simulink model "MJAUV_Maneuverability_model_V2"  (R2022b)
settings: Solver=ode4  StartTime=0.0  StopTime=50  FixedStep=0.0001  RelTol=1e-3  EnableMultiTasking=on
libraries: sharedutil x64, matrix_library x35
(part 3 of 5)

== system MJAUV_Maneuverability_model_V2/MJ-AUV Model & PropulsionSystem/Dynamics and Kinematics/Subsystem8/Damping forces1 ==
  nu_F : Inport
  Abs : Abs
  Create Diagonal Matrix : matrix_library/Create Diagonal Matrix
  Gain : Gain  Gain=-1
  Linear Damping Matrix : Constant  Value=DL
  Matrix Multiply : Product  Multiplication=Matrix(*)
  Product : Product  SaturateOnIntegerOverflow=on  OutDataTypeStr=Inherit: Same as first input
  Quadratic Damping Vector : Constant  Value=dQ_F
  Reshape1 : Reshape  OutputDimensionality=Column vector (2-D)
  Reshape2 : Reshape  OutputDimensionality=Column vector (2-D)  OutputDimensions=[6,6]
  Sum1 : Sum  Inputs=|++  SaturateOnIntegerOverflow=on
  D * nu_F : Outport  VectorParamsAs1DForOutWhenUnconnected=off
  wires:
  Reshape2/1 -> Product/1
  Reshape1/1 -> Matrix Multiply/2, Abs/1
  nu_F/1 -> Reshape1/1
  Linear Damping Matrix/1 -> Sum1/1
  Create Diagonal Matrix/1 -> Sum1/2
  Product/1 -> Create Diagonal Matrix/1
  Abs/1 -> Product/2  "abs(nu_F)"
  Quadratic Damping Vector/1 -> Reshape2/1  "dQ"
  Matrix Multiply/1 -> D * nu_F/1
  Sum1/1 -> Gain/1  "D"
  Gain/1 -> Matrix Multiply/1

== system MJAUV_Maneuverability_model_V2/MJ-AUV Model & PropulsionSystem/Dynamics and Kinematics/Subsystem8/Restoring forces1 ==
  eta_E : Inport
  3x3 Cross Product : sharedutil/3x3 Cross Product  aMode=aMode
  3x3 Cross Product1 : sharedutil/3x3 Cross Product  aMode=aMode
  E1(e) : Subsystem
  Gain : Gain  Gain=-1  SaturateOnIntegerOverflow=on  OutDataTypeStr=Inherit: Same as input  ParamDataTypeStr=Inherit: Same as input
  Matrix Multiply : Product  Multiplication=Matrix(*)
  Matrix Multiply1 : Product  Multiplication=Matrix(*)
  Mux : Mux  Inputs=2
  Selector : Selector  InputPortWidth=7  IndexOptions=Index vector (dialog)  Indices=[4 5 6 7]  OutputSizes=1
  Sum1 : Sum  Inputs=|++  SaturateOnIntegerOverflow=on
  Sum2 : Sum  Inputs=|++  SaturateOnIntegerOverflow=on
  Transpose : Math  Operator=transpose  SignedPower=on
  fBF_E : Constant  Value=[0;0;-B_F]
  fGF_E : Constant  Value=[0;0;W_F]
  rB_F : Constant  Value=rB_F
  rG_F : Constant  Value=rG_F
  g(eta_E)_T : Outport  VectorParamsAs1DForOutWhenUnconnected=off
  wires:
  E1(e)/1(E1) -> Transpose/1  "E1(e)"
  Transpose/1 -> Matrix Multiply/1, Matrix Multiply1/1  "E1(e)^T"
  fGF_E/1 -> Matrix Multiply/2
  fBF_E/1 -> Matrix Multiply1/2
  Matrix Multiply/1 -> Sum1/1, 3x3 Cross Product/2  "fG_F"
  Matrix Multiply1/1 -> Sum1/2, 3x3 Cross Product1/2  "fB_F"
  rG_F/1 -> 3x3 Cross Product/1
  Sum1/1 -> Mux/1  "fG_F + fB_F"
  3x3 Cross Product/1 -> Sum2/1  "rG_F x fG_F"
  3x3 Cross Product1/1 -> Sum2/2  "rB_F x fG_F"
  rB_F/1 -> 3x3 Cross Product1/1
  Sum2/1 -> Mux/2
  Mux/1 -> Gain/1
  Gain/1 -> g(eta_E)_T/1
  Selector/1 -> E1(e)/1(e)  "e"
  eta_E/1 -> Selector/1  "E1(e)"

== system MJAUV_Maneuverability_model_V2/MJ-AUV Model & PropulsionSystem/Dynamics and Kinematics/Subsystem8/Rigid-body Coriolis and centripetal matrix1 ==
  nu_F : Inport
  Gain : Gain  Gain=mF  SaturateOnIntegerOverflow=on  OutDataTypeStr=Inherit: Same as input  ParamDataTypeStr=Inherit: Same as input
  Gain1 : Gain  Gain=-mF  SaturateOnIntegerOverflow=on  OutDataTypeStr=Inherit: Same as input  ParamDataTypeStr=Inherit: Same as input
  Gain2 : Gain  Gain=-1  SaturateOnIntegerOverflow=on  OutDataTypeStr=Inherit: Same as input  ParamDataTypeStr=Inherit: Same as input
  Ib_F : Subsystem
  Matrix Concatenation : Concatenate  Mode=Multidimensional array
  Matrix Concatenation1 : Concatenate  Mode=Multidimensional array
  Matrix Concatenation2 : Concatenate  Mode=Multidimensional array  ConcatenateDimension=2
  Matrix Multiply : Product  Multiplication=Matrix(*)
  Matrix Multiply1 : Product  Multiplication=Matrix(*)
  Matrix Multiply2 : Product  Multiplication=Matrix(*)
  Selector : Selector  InputPortWidth=6  IndexOptions=Index vector (dialog)  Indices=[4 5 6]  OutputSizes=1
  Selector1 : Selector  InputPortWidth=6  IndexOptions=Index vector (dialog)  Indices=[1 2 3]  OutputSizes=1
  "Skew Symmetrical Operator " : Subsystem
  Skew Symmetrical Operator : Subsystem
  "Skew Symmetrical Operator " : Subsystem
  "Skew Symmetrical Operator  " : Subsystem
  Sum1 : Sum  Inputs=|++  SaturateOnIntegerOverflow=on
  Sum2 : Sum  Inputs=|-+  SaturateOnIntegerOverflow=on
  Zero matrix (3 x 3) : Constant  Value=zeros(3,3)
  rG_F : Constant  Value=rG_F
  CRB_F : Outport  VectorParamsAs1DForOutWhenUnconnected=off
  wires:
  Gain2/1 -> Matrix Concatenation1/2  "CRB(2,2)"
  Gain/1 -> Matrix Concatenation/2  "CRB(2,1)"
  rG_F/1 -> Ib_F/1(rG_F), "Skew Symmetrical Operator  "/1(v)  "rG_F"
  "Skew Symmetrical Operator "/1(S(V)) -> Gain2/1  "S(IO * nu_F2)"
  Selector1/1 -> Skew Symmetrical Operator/1(v)  "nu_F1"
  nu_F/1 -> Selector/1, Selector1/1
  Matrix Concatenation2/1 -> CRB_F/1
  Skew Symmetrical Operator/1(S(V)) -> Sum2/1, Sum1/1  "S(nu_F1)"
  Gain1/1 -> Matrix Concatenation1/1  "CRB(1,2)"
  Zero matrix (3 x 3)/1 -> Matrix Concatenation/1  "CRB(1,1)"
  Matrix Multiply2/1 -> "Skew Symmetrical Operator "/1(v)  "IO * nu_F2"
  Sum2/1 -> Gain/1
  Matrix Concatenation1/1 -> Matrix Concatenation2/2
  Selector/1 -> "Skew Symmetrical Operator "/1(v), Matrix Multiply2/2  "nu_F2"
  Matrix Multiply/1 -> Sum2/2  "S(rG_F) * S(nu_F2)"
  Ib_F/1(Ib_F) -> Matrix Multiply2/1
  Matrix Concatenation/1 -> Matrix Concatenation2/1
  "Skew Symmetrical Operator "/1(S(V)) -> Matrix Multiply/2, Matrix Multiply1/1  "S(nu_F2)"
  Sum1/1 -> Gain1/1
  Matrix Multiply1/1 -> Sum1/2  "S(nu_F2) * S(rG_F)"
  "Skew Symmetrical Operator  "/1(S(V)) -> Matrix Multiply/1, Matrix Multiply1/2  "S(rG_F)"

== system MJAUV_Maneuverability_model_V2/MJ-AUV Model & PropulsionSystem/Dynamics and Kinematics/Subsystem8/Subsystem1 ==
  eta_E_B : Inport
  Theta : Inport  Port=2
  Demux : Demux  Outputs=3
  Mux : Mux  Inputs=3
  Mux1 : Mux  Inputs=2
  Quaternion normalisation : Subsystem
  Quaternions to Euler Angles : Subsystem
  Selector : Selector  InputPortWidth=7  IndexOptions=Index vector (dialog)  Indices=[4 5 6 7]  OutputSizes=1
  Selector1 : Selector  InputPortWidth=3  IndexOptions=Index vector (dialog)  Indices=[1]  OutputSizes=1
  Selector2 : Selector  InputPortWidth=7  IndexOptions=Index vector (dialog)  Indices=[1 2 3]  OutputSizes=1
  Selector3 : Selector  InputPortWidth=3  IndexOptions=Index vector (dialog)  Indices=[2]  OutputSizes=1
  Selector4 : Selector  InputPortWidth=3  IndexOptions=Index vector (dialog)  Indices=[3]  OutputSizes=1
  Subsystem : Subsystem
  Subsystem1 : Subsystem
  Sum : Sum  Inputs=|||++++
  eta_E_T : Outport
  wires:
  eta_E_B/1 -> Selector2/1, Selector/1
  Selector/1 -> Quaternions to Euler Angles/1(Quaternions)  "e"
  Demux/2 -> Mux/2
  Demux/3 -> Sum/1
  Quaternions to Euler Angles/1(Euler Angles) -> Demux/1
  Subsystem/1(Quaternions) -> Mux1/2
  Selector1/1 -> Sum/2  "Theta1"
  Selector2/1 -> Mux1/1  "e"
  Mux/1 -> Subsystem/1("Euler Angles ")
  Demux/1 -> Mux/1
  Mux1/1 -> Quaternion normalisation/1(eta_E)
  Sum/1 -> Subsystem1/1(In2)
  Quaternion normalisation/1(eta_E (norm)) -> eta_E_T/1
  Theta/1 -> Selector4/1, Selector3/1, Selector1/1
  Selector3/1 -> Sum/3  "Theta2"
  Selector4/1 -> Sum/4  "Theta3"
  Subsystem1/1(Out1) -> Mux/3

== system MJAUV_Maneuverability_model_V2/MJ-AUV Model & PropulsionSystem/Dynamics and Kinematics/Subsystem9/M_B ==
  Add : Sum
  Constant1 : Constant  Value=rG_B
  Subsystem : Subsystem
  Subsystem1 : Subsystem
  M_B : Outport  VectorParamsAs1DForOutWhenUnconnected=off
  wires:
  Constant1/1 -> Subsystem1/1(rG_B)
  Subsystem1/1(MRB_B) -> Add/1
  Subsystem/1(MA_B) -> Add/2
  Add/1 -> M_B/1  "M_B"

== system MJAUV_Maneuverability_model_V2/MJ-AUV Model & PropulsionSystem/Dynamics and Kinematics/Subsystem9/M_F ==
  Add : Sum
  Constant1 : Constant  Value=rG_F
  Subsystem : Subsystem
  Subsystem1 : Subsystem
  M_F : Outport  VectorParamsAs1DForOutWhenUnconnected=off
  wires:
  Constant1/1 -> Subsystem1/1(rG_F)
  Subsystem1/1(MRB_F) -> Add/1
  Subsystem/1(MA_F) -> Add/2
  Add/1 -> M_F/1  "M_F"

== system MJAUV_Maneuverability_model_V2/MJ-AUV Model & PropulsionSystem/Dynamics and Kinematics/Subsystem9/M_S ==
  rG_S : Inport
  Add : Sum
  Subsystem : Subsystem
  Subsystem1 : Subsystem
  M_S : Outport  VectorParamsAs1DForOutWhenUnconnected=off
  wires:
  Add/1 -> M_S/1  "M_S"
  Subsystem/1(MA_S) -> Add/2
  Subsystem1/1(MRB_S) -> Add/1
  rG_S/1 -> Subsystem1/1(rG_S)

== system MJAUV_Maneuverability_model_V2/MJ-AUV Model & PropulsionSystem/Dynamics and Kinematics/Subsystem9/M_T ==
  Add : Sum
  Constant1 : Constant  Value=rG_T
  Subsystem : Subsystem
  Subsystem1 : Subsystem
  M_T : Outport  VectorParamsAs1DForOutWhenUnconnected=off
  wires:
  Add/1 -> M_T/1  "M_T"
  Subsystem/1(MA_T) -> Add/2
  Subsystem1/1(MRB_T) -> Add/1
  Constant1/1 -> Subsystem1/1(rG_T)

== system MJAUV_Maneuverability_model_V2/MJ-AUV Model & PropulsionSystem/Dynamics and Kinematics/Subsystem9/Subsystem5 ==
  Theta : Inport
  K : Subsystem
  K_B : Subsystem
  K_T : Subsystem
  Selector2 : Selector  InputPortWidth=3  IndexOptions=Index vector (dialog)  Indices=[1]  OutputSizes=1
  Selector3 : Selector  InputPortWidth=3  IndexOptions=Index vector (dialog)  Indices=[2]  OutputSizes=1
  Selector6 : Selector  InputPortWidth=3  IndexOptions=Index vector (dialog)  Indices=[3]  OutputSizes=1
  Transpose1 : matrix_library/Transpose
  Transpose2 : matrix_library/Transpose
  Transpose3 : matrix_library/Transpose
  "{B}->{S} Transformation" : Subsystem
  "{S}->{T} Transformation" : Subsystem
  "{T}->{F} Transformation" : Subsystem
  K_FT : Outport
  K_TS : Outport  Port=2
  K_SB : Outport  Port=3
  wires:
  Theta/1 -> Selector2/1, Selector3/1, Selector6/1
  K/1(K_FT) -> K_FT/1
  "{B}->{S} Transformation"/1(R(v)) -> Transpose3/1  "R_BS"
  Selector6/1 -> "{T}->{F} Transformation"/1(v)
  "{T}->{F} Transformation"/1(R(v)) -> Transpose1/1  "R_TF"
  Transpose3/1 -> K_B/1(R_SB)
  "{S}->{T} Transformation"/1(R(v)) -> Transpose2/1  "R_ST"
  Transpose2/1 -> K_T/1(R_TS)
  Selector2/1 -> "{B}->{S} Transformation"/1(v)
  Transpose1/1 -> K/1(R_FT)
  Selector3/1 -> "{S}->{T} Transformation"/1(v)
  K_B/1(K_SB) -> K_SB/1
  K_T/1(K_TS) -> K_TS/1

== system MJAUV_Maneuverability_model_V2/MJ-AUV Model & PropulsionSystem/Dynamics and Kinematics/6 DOF transformation/E1(e)/Skew Symmetrical Operator ==
  v : Inport
  Constant : Constant  Value=0
  Create 3x3 Matrix : sharedutil/Create 3x3 Matrix  aMode=aMode
  Demux : Demux  Outputs=3
      settings: DisplayOption=none
  Gain : Gain  Gain=-1  SaturateOnIntegerOverflow=on  OutDataTypeStr=Inherit: Same as input  ParamDataTypeStr=Inherit: Same as input
  Gain1 : Gain  Gain=-1  SaturateOnIntegerOverflow=on  OutDataTypeStr=Inherit: Same as input  ParamDataTypeStr=Inherit: Same as input
  Gain2 : Gain  Gain=-1  SaturateOnIntegerOverflow=on  OutDataTypeStr=Inherit: Same as input  ParamDataTypeStr=Inherit: Same as input
  S(V) : Outport  VectorParamsAs1DForOutWhenUnconnected=off
  wires:
  v/1 -> Demux/1
  Create 3x3 Matrix/1 -> S(V)/1
  Gain2/1 -> Create 3x3 Matrix/2  "-v(3)"
  Gain1/1 -> Create 3x3 Matrix/7  "-v(2)"
  Gain/1 -> Create 3x3 Matrix/6  "-v(1)"
  Demux/3 -> Create 3x3 Matrix/4, Gain2/1  "v(3)"
  Demux/2 -> Create 3x3 Matrix/3, Gain1/1  "v(2)"
  Demux/1 -> Create 3x3 Matrix/8, Gain/1  "v(1)"
  Constant/1 -> Create 3x3 Matrix/5, Create 3x3 Matrix/9, Create 3x3 Matrix/1

== system MJAUV_Maneuverability_model_V2/MJ-AUV Model & PropulsionSystem/Dynamics and Kinematics/6 DOF transformation/E2(e)/Skew Symmetrical Operator ==
  v : Inport
  Constant : Constant  Value=0
  Create 3x3 Matrix : sharedutil/Create 3x3 Matrix  aMode=aMode
  Demux : Demux  Outputs=3
      settings: DisplayOption=none
  Gain : Gain  Gain=-1  SaturateOnIntegerOverflow=on  OutDataTypeStr=Inherit: Same as input  ParamDataTypeStr=Inherit: Same as input
  Gain1 : Gain  Gain=-1  SaturateOnIntegerOverflow=on  OutDataTypeStr=Inherit: Same as input  ParamDataTypeStr=Inherit: Same as input
  Gain2 : Gain  Gain=-1  SaturateOnIntegerOverflow=on  OutDataTypeStr=Inherit: Same as input  ParamDataTypeStr=Inherit: Same as input
  S(V) : Outport  VectorParamsAs1DForOutWhenUnconnected=off
  wires:
  Constant/1 -> Create 3x3 Matrix/1, Create 3x3 Matrix/9, Create 3x3 Matrix/5
  Demux/1 -> Gain/1, Create 3x3 Matrix/8  "v(1)"
  Demux/2 -> Gain1/1, Create 3x3 Matrix/3  "v(2)"
  Demux/3 -> Gain2/1, Create 3x3 Matrix/4  "v(3)"
  Gain/1 -> Create 3x3 Matrix/6  "-v(1)"
  Gain1/1 -> Create 3x3 Matrix/7  "-v(2)"
  Gain2/1 -> Create 3x3 Matrix/2  "-v(3)"
  Create 3x3 Matrix/1 -> S(V)/1
  v/1 -> Demux/1

== system MJAUV_Maneuverability_model_V2/MJ-AUV Model & PropulsionSystem/Dynamics and Kinematics/Subsystem1/H_BS/Skew Symmetrical Operator  ==
  v : Inport
  Constant : Constant  Value=0
  Create 3x3 Matrix : sharedutil/Create 3x3 Matrix  aMode=aMode
  Demux : Demux  Outputs=3
      settings: DisplayOption=none
  Gain : Gain  Gain=-1  SaturateOnIntegerOverflow=on  OutDataTypeStr=Inherit: Same as input  ParamDataTypeStr=Inherit: Same as input
  Gain1 : Gain  Gain=-1  SaturateOnIntegerOverflow=on  OutDataTypeStr=Inherit: Same as input  ParamDataTypeStr=Inherit: Same as input
  Gain2 : Gain  Gain=-1  SaturateOnIntegerOverflow=on  OutDataTypeStr=Inherit: Same as input  ParamDataTypeStr=Inherit: Same as input
  S(V) : Outport  VectorParamsAs1DForOutWhenUnconnected=off
  wires:
  v/1 -> Demux/1
  Create 3x3 Matrix/1 -> S(V)/1
  Gain2/1 -> Create 3x3 Matrix/2  "-v(3)"
  Gain1/1 -> Create 3x3 Matrix/7  "-v(2)"
  Gain/1 -> Create 3x3 Matrix/6  "-v(1)"
  Demux/3 -> Create 3x3 Matrix/4, Gain2/1  "v(3)"
  Demux/2 -> Create 3x3 Matrix/3, Gain1/1  "v(2)"
  Demux/1 -> Create 3x3 Matrix/8, Gain/1  "v(1)"
  Constant/1 -> Create 3x3 Matrix/5, Create 3x3 Matrix/9, Create 3x3 Matrix/1

== system MJAUV_Maneuverability_model_V2/MJ-AUV Model & PropulsionSystem/Dynamics and Kinematics/Subsystem2/H_ST/Skew Symmetrical Operator  ==
  v : Inport
  Constant : Constant  Value=0
  Create 3x3 Matrix : sharedutil/Create 3x3 Matrix  aMode=aMode
  Demux : Demux  Outputs=3
      settings: DisplayOption=none
  Gain : Gain  Gain=-1  SaturateOnIntegerOverflow=on  OutDataTypeStr=Inherit: Same as input  ParamDataTypeStr=Inherit: Same as input
  Gain1 : Gain  Gain=-1  SaturateOnIntegerOverflow=on  OutDataTypeStr=Inherit: Same as input  ParamDataTypeStr=Inherit: Same as input
  Gain2 : Gain  Gain=-1  SaturateOnIntegerOverflow=on  OutDataTypeStr=Inherit: Same as input  ParamDataTypeStr=Inherit: Same as input
  S(V) : Outport  VectorParamsAs1DForOutWhenUnconnected=off
  wires:
  v/1 -> Demux/1
  Create 3x3 Matrix/1 -> S(V)/1
  Gain2/1 -> Create 3x3 Matrix/2  "-v(3)"
  Gain1/1 -> Create 3x3 Matrix/7  "-v(2)"
  Gain/1 -> Create 3x3 Matrix/6  "-v(1)"
  Demux/3 -> Create 3x3 Matrix/4, Gain2/1  "v(3)"
  Demux/2 -> Create 3x3 Matrix/3, Gain1/1  "v(2)"
  Demux/1 -> Create 3x3 Matrix/8, Gain/1  "v(1)"
  Constant/1 -> Create 3x3 Matrix/5, Create 3x3 Matrix/9, Create 3x3 Matrix/1

== system MJAUV_Maneuverability_model_V2/MJ-AUV Model & PropulsionSystem/Dynamics and Kinematics/Subsystem3/H_TF/Skew Symmetrical Operator  ==
  v : Inport
  Constant : Constant  Value=0
  Create 3x3 Matrix : sharedutil/Create 3x3 Matrix  aMode=aMode
  Demux : Demux  Outputs=3
      settings: DisplayOption=none
  Gain : Gain  Gain=-1  SaturateOnIntegerOverflow=on  OutDataTypeStr=Inherit: Same as input  ParamDataTypeStr=Inherit: Same as input
  Gain1 : Gain  Gain=-1  SaturateOnIntegerOverflow=on  OutDataTypeStr=Inherit: Same as input  ParamDataTypeStr=Inherit: Same as input
  Gain2 : Gain  Gain=-1  SaturateOnIntegerOverflow=on  OutDataTypeStr=Inherit: Same as input  ParamDataTypeStr=Inherit: Same as input
  S(V) : Outport  VectorParamsAs1DForOutWhenUnconnected=off
  wires:
  Constant/1 -> Create 3x3 Matrix/1, Create 3x3 Matrix/9, Create 3x3 Matrix/5
  Demux/1 -> Gain/1, Create 3x3 Matrix/8  "v(1)"
  Demux/2 -> Gain1/1, Create 3x3 Matrix/3  "v(2)"
  Demux/3 -> Gain2/1, Create 3x3 Matrix/4  "v(3)"
  Gain/1 -> Create 3x3 Matrix/6  "-v(1)"
  Gain1/1 -> Create 3x3 Matrix/7  "-v(2)"
  Gain2/1 -> Create 3x3 Matrix/2  "-v(3)"
  Create 3x3 Matrix/1 -> S(V)/1
  v/1 -> Demux/1

== system MJAUV_Maneuverability_model_V2/MJ-AUV Model & PropulsionSystem/Dynamics and Kinematics/Subsystem4/Added Mass Coriolis and centripetal matrix/Skew Symmetrical Operator ==
  v : Inport
  Constant : Constant  Value=0
  Create 3x3 Matrix : sharedutil/Create 3x3 Matrix  aMode=aMode
  Demux : Demux  Outputs=3
      settings: DisplayOption=none
  Gain : Gain  Gain=-1  SaturateOnIntegerOverflow=on  OutDataTypeStr=Inherit: Same as input  ParamDataTypeStr=Inherit: Same as input
  Gain1 : Gain  Gain=-1  SaturateOnIntegerOverflow=on  OutDataTypeStr=Inherit: Same as input  ParamDataTypeStr=Inherit: Same as input
  Gain2 : Gain  Gain=-1  SaturateOnIntegerOverflow=on  OutDataTypeStr=Inherit: Same as input  ParamDataTypeStr=Inherit: Same as input
  S(V) : Outport  VectorParamsAs1DForOutWhenUnconnected=off
  wires:
  Constant/1 -> Create 3x3 Matrix/1, Create 3x3 Matrix/9, Create 3x3 Matrix/5
  Demux/1 -> Gain/1, Create 3x3 Matrix/8  "v(1)"
  Demux/2 -> Gain1/1, Create 3x3 Matrix/3  "v(2)"
  Demux/3 -> Gain2/1, Create 3x3 Matrix/4  "v(3)"
  Gain/1 -> Create 3x3 Matrix/6  "-v(1)"
  Gain1/1 -> Create 3x3 Matrix/7  "-v(2)"
  Gain2/1 -> Create 3x3 Matrix/2  "-v(3)"
  Create 3x3 Matrix/1 -> S(V)/1
  v/1 -> Demux/1

== system MJAUV_Maneuverability_model_V2/MJ-AUV Model & PropulsionSystem/Dynamics and Kinematics/Subsystem4/Added Mass Coriolis and centripetal matrix/Skew Symmetrical Operator  ==
  v : Inport
  Constant : Constant  Value=0
  Create 3x3 Matrix : sharedutil/Create 3x3 Matrix  aMode=aMode
  Demux : Demux  Outputs=3
      settings: DisplayOption=none
  Gain : Gain  Gain=-1  SaturateOnIntegerOverflow=on  OutDataTypeStr=Inherit: Same as input  ParamDataTypeStr=Inherit: Same as input
  Gain1 : Gain  Gain=-1  SaturateOnIntegerOverflow=on  OutDataTypeStr=Inherit: Same as input  ParamDataTypeStr=Inherit: Same as input
  Gain2 : Gain  Gain=-1  SaturateOnIntegerOverflow=on  OutDataTypeStr=Inherit: Same as input  ParamDataTypeStr=Inherit: Same as input
  S(V) : Outport  VectorParamsAs1DForOutWhenUnconnected=off
  wires:
  v/1 -> Demux/1
  Create 3x3 Matrix/1 -> S(V)/1
  Gain2/1 -> Create 3x3 Matrix/2  "-v(3)"
  Gain1/1 -> Create 3x3 Matrix/7  "-v(2)"
  Gain/1 -> Create 3x3 Matrix/6  "-v(1)"
  Demux/3 -> Create 3x3 Matrix/4, Gain2/1  "v(3)"
  Demux/2 -> Create 3x3 Matrix/3, Gain1/1  "v(2)"
  Demux/1 -> Create 3x3 Matrix/8, Gain/1  "v(1)"
  Constant/1 -> Create 3x3 Matrix/5, Create 3x3 Matrix/9, Create 3x3 Matrix/1

== system MJAUV_Maneuverability_model_V2/MJ-AUV Model & PropulsionSystem/Dynamics and Kinematics/Subsystem4/Added Mass Coriolis and centripetal matrix/Subsystem ==
  Create Diagonal Matrix1 : matrix_library/Create Diagonal Matrix
  K_pdot_B : Constant  Value=0
  M_qdot_B : Constant  Value=(pi*rho*R^2*LB^3)/12
  Mux : Mux  Inputs=6
  N_rdot_B : Constant  Value=(pi*rho*R^2*LB^3)/12
  Reshape1 : Reshape  OutputDimensionality=Column vector (2-D)  OutputDimensions=[6,6]
  X_udot_B : Constant  Value=0.1*mB
  Y_vdot_B : Constant  Value=pi*rho*R*R*LB
  Z_wdot_B : Constant  Value=pi*rho*R^2*LB
  MA_B : Outport
  wires:
  Create Diagonal Matrix1/1 -> MA_B/1
  K_pdot_B/1 -> Mux/4
  N_rdot_B/1 -> Mux/6
  M_qdot_B/1 -> Mux/5
  X_udot_B/1 -> Mux/1
  Y_vdot_B/1 -> Mux/2
  Reshape1/1 -> Create Diagonal Matrix1/1
  Mux/1 -> Reshape1/1
  Z_wdot_B/1 -> Mux/3

== system MJAUV_Maneuverability_model_V2/MJ-AUV Model & PropulsionSystem/Dynamics and Kinematics/Subsystem4/Restoring forces/E1(e) ==
  e : Inport
  Gain : Gain  Gain=2  SaturateOnIntegerOverflow=on  OutDataTypeStr=Inherit: Same as input  ParamDataTypeStr=Inherit: Same as input
  "Gain " : Gain  Gain=2  SaturateOnIntegerOverflow=on  OutDataTypeStr=Inherit: Same as input  ParamDataTypeStr=Inherit: Same as input
  I (3x3) : Constant  Value=eye(3)
  Matrix Multiply : Product  Multiplication=Matrix(*)
  Product : Product  SaturateOnIntegerOverflow=on  OutDataTypeStr=Inherit: Same as first input
  Selector : Selector  InputPortWidth=4  IndexOptions=Index vector (dialog)  Indices=[1]  OutputSizes=1
  Selector1 : Selector  InputPortWidth=4  IndexOptions=Index vector (dialog)  Indices=[2 3 4]  OutputSizes=1
  Skew Symmetrical Operator : Subsystem
  Sum : Sum  Inputs=+++  SaturateOnIntegerOverflow=on
  E1 : Outport  VectorParamsAs1DForOutWhenUnconnected=off
  wires:
  e/1 -> Selector/1, Selector1/1
  Selector/1 -> "Gain "/1  "eta"
  Selector1/1 -> Skew Symmetrical Operator/1(v)  "eps"
  Skew Symmetrical Operator/1(S(V)) -> Matrix Multiply/1, Matrix Multiply/2, Product/2
  Matrix Multiply/1 -> Gain/1
  "Gain "/1 -> Product/1
  I (3x3)/1 -> Sum/1
  Product/1 -> Sum/2
  Gain/1 -> Sum/3
  Sum/1 -> E1/1

== system MJAUV_Maneuverability_model_V2/MJ-AUV Model & PropulsionSystem/Dynamics and Kinematics/Subsystem4/Rigid-body Coriolis and centripetal matrix/Skew Symmetrical Operator  ==
  v : Inport
  Constant : Constant  Value=0
  Create 3x3 Matrix : sharedutil/Create 3x3 Matrix  aMode=aMode
  Demux : Demux  Outputs=3
      settings: DisplayOption=none
  Gain : Gain  Gain=-1  SaturateOnIntegerOverflow=on  OutDataTypeStr=Inherit: Same as input  ParamDataTypeStr=Inherit: Same as input
  Gain1 : Gain  Gain=-1  SaturateOnIntegerOverflow=on  OutDataTypeStr=Inherit: Same as input  ParamDataTypeStr=Inherit: Same as input
  Gain2 : Gain  Gain=-1  SaturateOnIntegerOverflow=on  OutDataTypeStr=Inherit: Same as input  ParamDataTypeStr=Inherit: Same as input
  S(V) : Outport  VectorParamsAs1DForOutWhenUnconnected=off
  wires:
  v/1 -> Demux/1
  Create 3x3 Matrix/1 -> S(V)/1
  Gain2/1 -> Create 3x3 Matrix/2  "-v(3)"
  Gain1/1 -> Create 3x3 Matrix/7  "-v(2)"
  Gain/1 -> Create 3x3 Matrix/6  "-v(1)"
  Demux/3 -> Create 3x3 Matrix/4, Gain2/1  "v(3)"
  Demux/2 -> Create 3x3 Matrix/3, Gain1/1  "v(2)"
  Demux/1 -> Create 3x3 Matrix/8, Gain/1  "v(1)"
  Constant/1 -> Create 3x3 Matrix/5, Create 3x3 Matrix/9, Create 3x3 Matrix/1

== system MJAUV_Maneuverability_model_V2/MJ-AUV Model & PropulsionSystem/Dynamics and Kinematics/Subsystem4/Rigid-body Coriolis and centripetal matrix/Skew Symmetrical Operator ==
  v : Inport
  Constant : Constant  Value=0
  Create 3x3 Matrix : sharedutil/Create 3x3 Matrix  aMode=aMode
  Demux : Demux  Outputs=3
      settings: DisplayOption=none
  Gain : Gain  Gain=-1  SaturateOnIntegerOverflow=on  OutDataTypeStr=Inherit: Same as input  ParamDataTypeStr=Inherit: Same as input
  Gain1 : Gain  Gain=-1  SaturateOnIntegerOverflow=on  OutDataTypeStr=Inherit: Same as input  ParamDataTypeStr=Inherit: Same as input
  Gain2 : Gain  Gain=-1  SaturateOnIntegerOverflow=on  OutDataTypeStr=Inherit: Same as input  ParamDataTypeStr=Inherit: Same as input
  S(V) : Outport  VectorParamsAs1DForOutWhenUnconnected=off
  wires:
  v/1 -> Demux/1
  Create 3x3 Matrix/1 -> S(V)/1
  Gain2/1 -> Create 3x3 Matrix/2  "-v(3)"
  Gain1/1 -> Create 3x3 Matrix/7  "-v(2)"
  Gain/1 -> Create 3x3 Matrix/6  "-v(1)"
  Demux/3 -> Create 3x3 Matrix/4, Gain2/1  "v(3)"
  Demux/2 -> Create 3x3 Matrix/3, Gain1/1  "v(2)"
  Demux/1 -> Create 3x3 Matrix/8, Gain/1  "v(1)"
  Constant/1 -> Create 3x3 Matrix/5, Create 3x3 Matrix/9, Create 3x3 Matrix/1

== system MJAUV_Maneuverability_model_V2/MJ-AUV Model & PropulsionSystem/Dynamics and Kinematics/Subsystem4/Rigid-body Coriolis and centripetal matrix/Skew Symmetrical Operator  ==
  v : Inport
  Constant : Constant  Value=0
  Create 3x3 Matrix : sharedutil/Create 3x3 Matrix  aMode=aMode
  Demux : Demux  Outputs=3
      settings: DisplayOption=none
  Gain : Gain  Gain=-1  SaturateOnIntegerOverflow=on  OutDataTypeStr=Inherit: Same as input  ParamDataTypeStr=Inherit: Same as input
  Gain1 : Gain  Gain=-1  SaturateOnIntegerOverflow=on  OutDataTypeStr=Inherit: Same as input  ParamDataTypeStr=Inherit: Same as input
  Gain2 : Gain  Gain=-1  SaturateOnIntegerOverflow=on  OutDataTypeStr=Inherit: Same as input  ParamDataTypeStr=Inherit: Same as input
  S(V) : Outport  VectorParamsAs1DForOutWhenUnconnected=off
  wires:
  Constant/1 -> Create 3x3 Matrix/1, Create 3x3 Matrix/9, Create 3x3 Matrix/5
  Demux/1 -> Gain/1, Create 3x3 Matrix/8  "v(1)"
  Demux/2 -> Gain1/1, Create 3x3 Matrix/3  "v(2)"
  Demux/3 -> Gain2/1, Create 3x3 Matrix/4  "v(3)"
  Gain/1 -> Create 3x3 Matrix/6  "-v(1)"
  Gain1/1 -> Create 3x3 Matrix/7  "-v(2)"
  Gain2/1 -> Create 3x3 Matrix/2  "-v(3)"
  Create 3x3 Matrix/1 -> S(V)/1
  v/1 -> Demux/1

== system MJAUV_Maneuverability_model_V2/MJ-AUV Model & PropulsionSystem/Dynamics and Kinematics/Subsystem4/Rigid-body Coriolis and centripetal matrix/Skew Symmetrical Operator   ==
  v : Inport
  Constant : Constant  Value=0
  Create 3x3 Matrix : sharedutil/Create 3x3 Matrix  aMode=aMode
  Demux : Demux  Outputs=3
      settings: DisplayOption=none
  Gain : Gain  Gain=-1  SaturateOnIntegerOverflow=on  OutDataTypeStr=Inherit: Same as input  ParamDataTypeStr=Inherit: Same as input
  Gain1 : Gain  Gain=-1  SaturateOnIntegerOverflow=on  OutDataTypeStr=Inherit: Same as input  ParamDataTypeStr=Inherit: Same as input
  Gain2 : Gain  Gain=-1  SaturateOnIntegerOverflow=on  OutDataTypeStr=Inherit: Same as input  ParamDataTypeStr=Inherit: Same as input
  S(V) : Outport  VectorParamsAs1DForOutWhenUnconnected=off
  wires:
  v/1 -> Demux/1
  Create 3x3 Matrix/1 -> S(V)/1
  Gain2/1 -> Create 3x3 Matrix/2  "-v(3)"
  Gain1/1 -> Create 3x3 Matrix/7  "-v(2)"
  Gain/1 -> Create 3x3 Matrix/6  "-v(1)"
  Demux/3 -> Create 3x3 Matrix/4, Gain2/1  "v(3)"
  Demux/2 -> Create 3x3 Matrix/3, Gain1/1  "v(2)"
  Demux/1 -> Create 3x3 Matrix/8, Gain/1  "v(1)"
  Constant/1 -> Create 3x3 Matrix/5, Create 3x3 Matrix/9, Create 3x3 Matrix/1

== system MJAUV_Maneuverability_model_V2/MJ-AUV Model & PropulsionSystem/Dynamics and Kinematics/Subsystem4/Rigid-body Coriolis and centripetal matrix/Subsystem ==
  rG_B : Inport
  Add : Sum
  Constant2 : Constant  Value=IB
  Gain5 : Gain  Gain=-mB
  Matrix Multiply4 : Product  Multiplication=Matrix(*)
  Skew Symmetrical Operator1 : Subsystem
  Ib_B : Outport
  wires:
  rG_B/1 -> Skew Symmetrical Operator1/1(v)  "rG_B"
  Constant2/1 -> Add/1
  Gain5/1 -> Add/2
  Matrix Multiply4/1 -> Gain5/1
  Skew Symmetrical Operator1/1(S(V)) -> Matrix Multiply4/1, Matrix Multiply4/2  "skewsymm(rG_B)"
  Add/1 -> Ib_B/1  "Ib_B"

== system MJAUV_Maneuverability_model_V2/MJ-AUV Model & PropulsionSystem/Dynamics and Kinematics/Subsystem5/K/Skew Symmetrical Operator  ==
  v : Inport
  Constant : Constant  Value=0
  Create 3x3 Matrix : sharedutil/Create 3x3 Matrix  aMode=aMode
  Demux : Demux  Outputs=3
      settings: DisplayOption=none
  Gain : Gain  Gain=-1  SaturateOnIntegerOverflow=on  OutDataTypeStr=Inherit: Same as input  ParamDataTypeStr=Inherit: Same as input
  Gain1 : Gain  Gain=-1  SaturateOnIntegerOverflow=on  OutDataTypeStr=Inherit: Same as input  ParamDataTypeStr=Inherit: Same as input
  Gain2 : Gain  Gain=-1  SaturateOnIntegerOverflow=on  OutDataTypeStr=Inherit: Same as input  ParamDataTypeStr=Inherit: Same as input
  S(V) : Outport  VectorParamsAs1DForOutWhenUnconnected=off
  wires:
  Constant/1 -> Create 3x3 Matrix/1, Create 3x3 Matrix/9, Create 3x3 Matrix/5
  Demux/1 -> Gain/1, Create 3x3 Matrix/8  "v(1)"
  Demux/2 -> Gain1/1, Create 3x3 Matrix/3  "v(2)"
  Demux/3 -> Gain2/1, Create 3x3 Matrix/4  "v(3)"
  Gain/1 -> Create 3x3 Matrix/6  "-v(1)"
  Gain1/1 -> Create 3x3 Matrix/7  "-v(2)"
  Gain2/1 -> Create 3x3 Matrix/2  "-v(3)"
  Create 3x3 Matrix/1 -> S(V)/1
  v/1 -> Demux/1

== system MJAUV_Maneuverability_model_V2/MJ-AUV Model & PropulsionSystem/Dynamics and Kinematics/Subsystem5/K_B/Skew Symmetrical Operator  ==
  v : Inport
  Constant : Constant  Value=0
  Create 3x3 Matrix : sharedutil/Create 3x3 Matrix  aMode=aMode
  Demux : Demux  Outputs=3
      settings: DisplayOption=none
  Gain : Gain  Gain=-1  SaturateOnIntegerOverflow=on  OutDataTypeStr=Inherit: Same as input  ParamDataTypeStr=Inherit: Same as input
  Gain1 : Gain  Gain=-1  SaturateOnIntegerOverflow=on  OutDataTypeStr=Inherit: Same as input  ParamDataTypeStr=Inherit: Same as input
  Gain2 : Gain  Gain=-1  SaturateOnIntegerOverflow=on  OutDataTypeStr=Inherit: Same as input  ParamDataTypeStr=Inherit: Same as input
  S(V) : Outport  VectorParamsAs1DForOutWhenUnconnected=off
  wires:
  v/1 -> Demux/1
  Create 3x3 Matrix/1 -> S(V)/1
  Gain2/1 -> Create 3x3 Matrix/2  "-v(3)"
  Gain1/1 -> Create 3x3 Matrix/7  "-v(2)"
  Gain/1 -> Create 3x3 Matrix/6  "-v(1)"
  Demux/3 -> Create 3x3 Matrix/4, Gain2/1  "v(3)"
  Demux/2 -> Create 3x3 Matrix/3, Gain1/1  "v(2)"
  Demux/1 -> Create 3x3 Matrix/8, Gain/1  "v(1)"
  Constant/1 -> Create 3x3 Matrix/5, Create 3x3 Matrix/9, Create 3x3 Matrix/1

== system MJAUV_Maneuverability_model_V2/MJ-AUV Model & PropulsionSystem/Dynamics and Kinematics/Subsystem5/K_T/Skew Symmetrical Operator  ==
  v : Inport
  Constant : Constant  Value=0
  Create 3x3 Matrix : sharedutil/Create 3x3 Matrix  aMode=aMode
  Demux : Demux  Outputs=3
      settings: DisplayOption=none
  Gain : Gain  Gain=-1  SaturateOnIntegerOverflow=on  OutDataTypeStr=Inherit: Same as input  ParamDataTypeStr=Inherit: Same as input
  Gain1 : Gain  Gain=-1  SaturateOnIntegerOverflow=on  OutDataTypeStr=Inherit: Same as input  ParamDataTypeStr=Inherit: Same as input
  Gain2 : Gain  Gain=-1  SaturateOnIntegerOverflow=on  OutDataTypeStr=Inherit: Same as input  ParamDataTypeStr=Inherit: Same as input
  S(V) : Outport  VectorParamsAs1DForOutWhenUnconnected=off
  wires:
  v/1 -> Demux/1
  Create 3x3 Matrix/1 -> S(V)/1
  Gain2/1 -> Create 3x3 Matrix/2  "-v(3)"
  Gain1/1 -> Create 3x3 Matrix/7  "-v(2)"
  Gain/1 -> Create 3x3 Matrix/6  "-v(1)"
  Demux/3 -> Create 3x3 Matrix/4, Gain2/1  "v(3)"
  Demux/2 -> Create 3x3 Matrix/3, Gain1/1  "v(2)"
  Demux/1 -> Create 3x3 Matrix/8, Gain/1  "v(1)"
  Constant/1 -> Create 3x3 Matrix/5, Create 3x3 Matrix/9, Create 3x3 Matrix/1

== system MJAUV_Maneuverability_model_V2/MJ-AUV Model & PropulsionSystem/Dynamics and Kinematics/Subsystem6/Added Mass Coriolis and centripetal matrix1/Skew Symmetrical Operator ==
  v : Inport
  Constant : Constant  Value=0
  Create 3x3 Matrix : sharedutil/Create 3x3 Matrix  aMode=aMode
  Demux : Demux  Outputs=3
      settings: DisplayOption=none
  Gain : Gain  Gain=-1  SaturateOnIntegerOverflow=on  OutDataTypeStr=Inherit: Same as input  ParamDataTypeStr=Inherit: Same as input
  Gain1 : Gain  Gain=-1  SaturateOnIntegerOverflow=on  OutDataTypeStr=Inherit: Same as input  ParamDataTypeStr=Inherit: Same as input
  Gain2 : Gain  Gain=-1  SaturateOnIntegerOverflow=on  OutDataTypeStr=Inherit: Same as input  ParamDataTypeStr=Inherit: Same as input
  S(V) : Outport  VectorParamsAs1DForOutWhenUnconnected=off
  wires:
  v/1 -> Demux/1
  Create 3x3 Matrix/1 -> S(V)/1
  Gain2/1 -> Create 3x3 Matrix/2  "-v(3)"
  Gain1/1 -> Create 3x3 Matrix/7  "-v(2)"
  Gain/1 -> Create 3x3 Matrix/6  "-v(1)"
  Demux/3 -> Create 3x3 Matrix/4, Gain2/1  "v(3)"
  Demux/2 -> Create 3x3 Matrix/3, Gain1/1  "v(2)"
  Demux/1 -> Create 3x3 Matrix/8, Gain/1  "v(1)"
  Constant/1 -> Create 3x3 Matrix/5, Create 3x3 Matrix/9, Create 3x3 Matrix/1

== system MJAUV_Maneuverability_model_V2/MJ-AUV Model & PropulsionSystem/Dynamics and Kinematics/Subsystem6/Added Mass Coriolis and centripetal matrix1/Skew Symmetrical Operator  ==
  v : Inport
  Constant : Constant  Value=0
  Create 3x3 Matrix : sharedutil/Create 3x3 Matrix  aMode=aMode
  Demux : Demux  Outputs=3
      settings: DisplayOption=none
  Gain : Gain  Gain=-1  SaturateOnIntegerOverflow=on  OutDataTypeStr=Inherit: Same as input  ParamDataTypeStr=Inherit: Same as input
  Gain1 : Gain  Gain=-1  SaturateOnIntegerOverflow=on  OutDataTypeStr=Inherit: Same as input  ParamDataTypeStr=Inherit: Same as input
  Gain2 : Gain  Gain=-1  SaturateOnIntegerOverflow=on  OutDataTypeStr=Inherit: Same as input  ParamDataTypeStr=Inherit: Same as input
  S(V) : Outport  VectorParamsAs1DForOutWhenUnconnected=off
  wires:
  Constant/1 -> Create 3x3 Matrix/1, Create 3x3 Matrix/9, Create 3x3 Matrix/5
  Demux/1 -> Gain/1, Create 3x3 Matrix/8  "v(1)"
  Demux/2 -> Gain1/1, Create 3x3 Matrix/3  "v(2)"
  Demux/3 -> Gain2/1, Create 3x3 Matrix/4  "v(3)"
  Gain/1 -> Create 3x3 Matrix/6  "-v(1)"
  Gain1/1 -> Create 3x3 Matrix/7  "-v(2)"
  Gain2/1 -> Create 3x3 Matrix/2  "-v(3)"
  Create 3x3 Matrix/1 -> S(V)/1
  v/1 -> Demux/1

== system MJAUV_Maneuverability_model_V2/MJ-AUV Model & PropulsionSystem/Dynamics and Kinematics/Subsystem6/Added Mass Coriolis and centripetal matrix1/Subsystem ==
  Create Diagonal Matrix1 : matrix_library/Create Diagonal Matrix
  K_pdot_S : Constant  Value=0
  M_qdot_S : Constant  Value=(pi*rho*R^2*LS^3)/12
  Mux : Mux  Inputs=6
  N_rdot_S : Constant  Value=(pi*rho*R^2*LS^3)/12
  Reshape1 : Reshape  OutputDimensionality=Column vector (2-D)  OutputDimensions=[6,6]
  X_udot_S : Constant  Value=0.1*mS
  Y_vdot_S : Constant  Value=pi*rho*R*R*LS
  Z_wdot_S : Constant  Value=pi*rho*R^2*LS
  MA_S : Outport
  wires:
  Z_wdot_S/1 -> Mux/3
  Mux/1 -> Reshape1/1
  Reshape1/1 -> Create Diagonal Matrix1/1
  Y_vdot_S/1 -> Mux/2
  X_udot_S/1 -> Mux/1
  M_qdot_S/1 -> Mux/5
  N_rdot_S/1 -> Mux/6
  K_pdot_S/1 -> Mux/4
  Create Diagonal Matrix1/1 -> MA_S/1

== system MJAUV_Maneuverability_model_V2/MJ-AUV Model & PropulsionSystem/Dynamics and Kinematics/Subsystem6/Restoring forces1/E1(e) ==
  e : Inport
  Gain : Gain  Gain=2  SaturateOnIntegerOverflow=on  OutDataTypeStr=Inherit: Same as input  ParamDataTypeStr=Inherit: Same as input
  "Gain " : Gain  Gain=2  SaturateOnIntegerOverflow=on  OutDataTypeStr=Inherit: Same as input  ParamDataTypeStr=Inherit: Same as input
  I (3x3) : Constant  Value=eye(3)
  Matrix Multiply : Product  Multiplication=Matrix(*)
  Product : Product  SaturateOnIntegerOverflow=on  OutDataTypeStr=Inherit: Same as first input
  Selector : Selector  InputPortWidth=4  IndexOptions=Index vector (dialog)  Indices=[1]  OutputSizes=1
  Selector1 : Selector  InputPortWidth=4  IndexOptions=Index vector (dialog)  Indices=[2 3 4]  OutputSizes=1
  Skew Symmetrical Operator : Subsystem
  Sum : Sum  Inputs=+++  SaturateOnIntegerOverflow=on
  E1 : Outport  VectorParamsAs1DForOutWhenUnconnected=off
  wires:
  Sum/1 -> E1/1
  Gain/1 -> Sum/3
  Product/1 -> Sum/2
  I (3x3)/1 -> Sum/1
  "Gain "/1 -> Product/1
  Matrix Multiply/1 -> Gain/1
  Skew Symmetrical Operator/1(S(V)) -> Product/2, Matrix Multiply/2, Matrix Multiply/1
  Selector1/1 -> Skew Symmetrical Operator/1(v)  "eps"
  Selector/1 -> "Gain "/1  "eta"
  e/1 -> Selector1/1, Selector/1

== system MJAUV_Maneuverability_model_V2/MJ-AUV Model & PropulsionSystem/Dynamics and Kinematics/Subsystem6/Rigid-body Coriolis and centripetal matrix1/Skew Symmetrical Operator  ==
  v : Inport
  Constant : Constant  Value=0
  Create 3x3 Matrix : sharedutil/Create 3x3 Matrix  aMode=aMode
  Demux : Demux  Outputs=3
      settings: DisplayOption=none
  Gain : Gain  Gain=-1  SaturateOnIntegerOverflow=on  OutDataTypeStr=Inherit: Same as input  ParamDataTypeStr=Inherit: Same as input
  Gain1 : Gain  Gain=-1  SaturateOnIntegerOverflow=on  OutDataTypeStr=Inherit: Same as input  ParamDataTypeStr=Inherit: Same as input
  Gain2 : Gain  Gain=-1  SaturateOnIntegerOverflow=on  OutDataTypeStr=Inherit: Same as input  ParamDataTypeStr=Inherit: Same as input
  S(V) : Outport  VectorParamsAs1DForOutWhenUnconnected=off
  wires:
  Constant/1 -> Create 3x3 Matrix/1, Create 3x3 Matrix/9, Create 3x3 Matrix/5
  Demux/1 -> Gain/1, Create 3x3 Matrix/8  "v(1)"
  Demux/2 -> Gain1/1, Create 3x3 Matrix/3  "v(2)"
  Demux/3 -> Gain2/1, Create 3x3 Matrix/4  "v(3)"
  Gain/1 -> Create 3x3 Matrix/6  "-v(1)"
  Gain1/1 -> Create 3x3 Matrix/7  "-v(2)"
  Gain2/1 -> Create 3x3 Matrix/2  "-v(3)"
  Create 3x3 Matrix/1 -> S(V)/1
  v/1 -> Demux/1

== system MJAUV_Maneuverability_model_V2/MJ-AUV Model & PropulsionSystem/Dynamics and Kinematics/Subsystem6/Rigid-body Coriolis and centripetal matrix1/Skew Symmetrical Operator ==
  v : Inport
  Constant : Constant  Value=0
  Create 3x3 Matrix : sharedutil/Create 3x3 Matrix  aMode=aMode
  Demux : Demux  Outputs=3
      settings: DisplayOption=none
  Gain : Gain  Gain=-1  SaturateOnIntegerOverflow=on  OutDataTypeStr=Inherit: Same as input  ParamDataTypeStr=Inherit: Same as input
  Gain1 : Gain  Gain=-1  SaturateOnIntegerOverflow=on  OutDataTypeStr=Inherit: Same as input  ParamDataTypeStr=Inherit: Same as input
  Gain2 : Gain  Gain=-1  SaturateOnIntegerOverflow=on  OutDataTypeStr=Inherit: Same as input  ParamDataTypeStr=Inherit: Same as input
  S(V) : Outport  VectorParamsAs1DForOutWhenUnconnected=off
  wires:
  Constant/1 -> Create 3x3 Matrix/1, Create 3x3 Matrix/9, Create 3x3 Matrix/5
  Demux/1 -> Gain/1, Create 3x3 Matrix/8  "v(1)"
  Demux/2 -> Gain1/1, Create 3x3 Matrix/3  "v(2)"
  Demux/3 -> Gain2/1, Create 3x3 Matrix/4  "v(3)"
  Gain/1 -> Create 3x3 Matrix/6  "-v(1)"
  Gain1/1 -> Create 3x3 Matrix/7  "-v(2)"
  Gain2/1 -> Create 3x3 Matrix/2  "-v(3)"
  Create 3x3 Matrix/1 -> S(V)/1
  v/1 -> Demux/1

== system MJAUV_Maneuverability_model_V2/MJ-AUV Model & PropulsionSystem/Dynamics and Kinematics/Subsystem6/Rigid-body Coriolis and centripetal matrix1/Skew Symmetrical Operator  ==
  v : Inport
  Constant : Constant  Value=0
  Create 3x3 Matrix : sharedutil/Create 3x3 Matrix  aMode=aMode
  Demux : Demux  Outputs=3
      settings: DisplayOption=none
  Gain : Gain  Gain=-1  SaturateOnIntegerOverflow=on  OutDataTypeStr=Inherit: Same as input  ParamDataTypeStr=Inherit: Same as input
  Gain1 : Gain  Gain=-1  SaturateOnIntegerOverflow=on  OutDataTypeStr=Inherit: Same as input  ParamDataTypeStr=Inherit: Same as input
  Gain2 : Gain  Gain=-1  SaturateOnIntegerOverflow=on  OutDataTypeStr=Inherit: Same as input  ParamDataTypeStr=Inherit: Same as input
  S(V) : Outport  VectorParamsAs1DForOutWhenUnconnected=off
  wires:
  v/1 -> Demux/1
  Create 3x3 Matrix/1 -> S(V)/1
  Gain2/1 -> Create 3x3 Matrix/2  "-v(3)"
  Gain1/1 -> Create 3x3 Matrix/7  "-v(2)"
  Gain/1 -> Create 3x3 Matrix/6  "-v(1)"
  Demux/3 -> Create 3x3 Matrix/4, Gain2/1  "v(3)"
  Demux/2 -> Create 3x3 Matrix/3, Gain1/1  "v(2)"
  Demux/1 -> Create 3x3 Matrix/8, Gain/1  "v(1)"
  Constant/1 -> Create 3x3 Matrix/5, Create 3x3 Matrix/9, Create 3x3 Matrix/1

== system MJAUV_Maneuverability_model_V2/MJ-AUV Model & PropulsionSystem/Dynamics and Kinematics/Subsystem6/Rigid-body Coriolis and centripetal matrix1/Skew Symmetrical Operator   ==
  v : Inport
  Constant : Constant  Value=0
  Create 3x3 Matrix : sharedutil/Create 3x3 Matrix  aMode=aMode
  Demux : Demux  Outputs=3
      settings: DisplayOption=none
  Gain : Gain  Gain=-1  SaturateOnIntegerOverflow=on  OutDataTypeStr=Inherit: Same as input  ParamDataTypeStr=Inherit: Same as input
  Gain1 : Gain  Gain=-1  SaturateOnIntegerOverflow=on  OutDataTypeStr=Inherit: Same as input  ParamDataTypeStr=Inherit: Same as input
  Gain2 : Gain  Gain=-1  SaturateOnIntegerOverflow=on  OutDataTypeStr=Inherit: Same as input  ParamDataTypeStr=Inherit: Same as input
  S(V) : Outport  VectorParamsAs1DForOutWhenUnconnected=off
  wires:
  Constant/1 -> Create 3x3 Matrix/1, Create 3x3 Matrix/9, Create 3x3 Matrix/5
  Demux/1 -> Gain/1, Create 3x3 Matrix/8  "v(1)"
  Demux/2 -> Gain1/1, Create 3x3 Matrix/3  "v(2)"
  Demux/3 -> Gain2/1, Create 3x3 Matrix/4  "v(3)"
  Gain/1 -> Create 3x3 Matrix/6  "-v(1)"
  Gain1/1 -> Create 3x3 Matrix/7  "-v(2)"
  Gain2/1 -> Create 3x3 Matrix/2  "-v(3)"
  Create 3x3 Matrix/1 -> S(V)/1
  v/1 -> Demux/1

== system MJAUV_Maneuverability_model_V2/MJ-AUV Model & PropulsionSystem/Dynamics and Kinematics/Subsystem6/Rigid-body Coriolis and centripetal matrix1/Subsystem ==
  rG_S : Inport
  Add : Sum
  Constant2 : Constant  Value=IS
  Gain5 : Gain  Gain=-mS
  Matrix Multiply4 : Product  Multiplication=Matrix(*)
  Skew Symmetrical Operator1 : Subsystem
  Ib_S : Outport
  wires:
  rG_S/1 -> Skew Symmetrical Operator1/1(v)  "rG_S"
  Constant2/1 -> Add/1
  Gain5/1 -> Add/2
  Matrix Multiply4/1 -> Gain5/1
  Skew Symmetrical Operator1/1(S(V)) -> Matrix Multiply4/1, Matrix Multiply4/2  "skewsymm(rG_S)"
  Add/1 -> Ib_S/1  "Ib_S"

== system MJAUV_Maneuverability_model_V2/MJ-AUV Model & PropulsionSystem/Dynamics and Kinematics/Subsystem6/Subsystem1/Quaternion normalisation ==
  eta_E : Inport
  Mux : Mux  Inputs=2
  Product : Product  Inputs=*/  SaturateOnIntegerOverflow=on  OutDataTypeStr=Inherit: Same as first input
  Reshape : Reshape  OutputDimensionality=Column vector (2-D)
  Selector : Selector  InputPortWidth=7  IndexOptions=Index vector (dialog)  Indices=[1 2 3]  OutputSizes=1
  Selector1 : Selector  InputPortWidth=7  IndexOptions=Index vector (dialog)  Indices=[4 5 6 7]  OutputSizes=1
  norm 1x4 vector : Subsystem
  eta_E (norm) : Outport  VectorParamsAs1DForOutWhenUnconnected=off
  wires:
  norm 1x4 vector/1(norm) -> Product/2
  Reshape/1 -> eta_E (norm)/1
  Mux/1 -> Reshape/1
  Product/1 -> Mux/2
  Selector/1 -> Mux/1
  Selector1/1 -> Product/1, norm 1x4 vector/1(Inport)
  eta_E/1 -> Selector/1, Selector1/1  "eta_E"

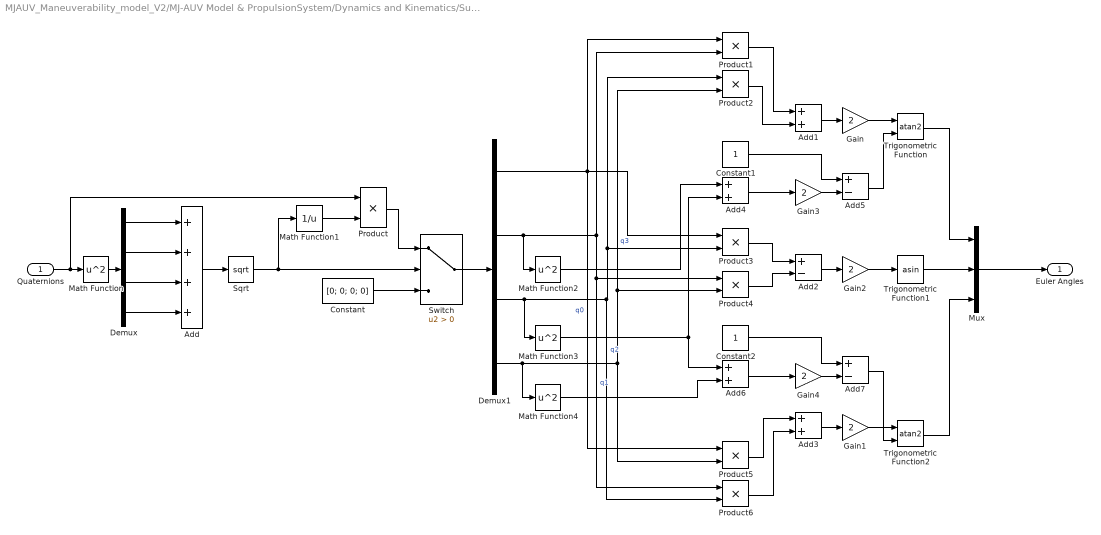
== system MJAUV_Maneuverability_model_V2/MJ-AUV Model & PropulsionSystem/Dynamics and Kinematics/Subsystem6/Subsystem1/Quaternions to Euler Angles ==
  Quaternions : Inport
  Add : Sum  Inputs=4
  Add{1,3..4,6} (4 alike) : Sum
  Add2 : Sum  Inputs=+-
  Add5 : Sum  Inputs=+-
  Add7 : Sum  Inputs=+-
  Constant : Constant  Value=[0; 0; 0; 0]
  Constant1 : Constant
  Constant2 : Constant
  Demux : Demux
  Demux1 : Demux
  Gain{,1..4} (5 alike) : Gain  Gain=2
  Math Function{,2..4} (4 alike) : Math  Operator=square  SignedPower=on
  Math Function1 : Math  Operator=reciprocal  SignedPower=on
  Mux : Mux  Inputs=3
  Product{,1..6} (7 alike) : Product
  Sqrt : Sqrt
  Switch : Switch  Criteria=u2 > Threshold  SaturateOnIntegerOverflow=off  InputSameDT=off
  Trigonometric Function : Trigonometry  Operator=atan2
  Trigonometric Function1 : Trigonometry  Operator=asin
  Trigonometric Function2 : Trigonometry  Operator=atan2
  Euler Angles : Outport  VectorParamsAs1DForOutWhenUnconnected=off
  wires:
  Quaternions/1 -> Product/1, Math Function/1
  Add/1 -> Sqrt/1
  Sqrt/1 -> Math Function1/1, Switch/2
  Constant/1 -> Switch/3
  Math Function1/1 -> Product/2
  Product/1 -> Switch/1
  Switch/1 -> Demux1/1
  Demux1/1 -> Product5/1, Product3/1, Product1/1  "q0"
  Demux1/2 -> Product6/1, Product4/1, Product1/2, Math Function2/1  "q1"
  Demux1/3 -> Product6/2, Product3/2, Product2/1, Math Function3/1  "q2"
  Demux1/4 -> Product5/2, Product4/2, Product2/2, Math Function4/1  "q3"
  Trigonometric Function1/1 -> Mux/2
  Mux/1 -> Euler Angles/1
  Trigonometric Function/1 -> Mux/1
  Trigonometric Function2/1 -> Mux/3
  Gain/1 -> Trigonometric Function/1
  Gain1/1 -> Trigonometric Function2/1
  Gain2/1 -> Trigonometric Function1/1
  Add1/1 -> Gain/1
  Add2/1 -> Gain2/1
  Add3/1 -> Gain1/1
  Product3/1 -> Add2/1
  Product4/1 -> Add2/2
  Product5/1 -> Add3/1
  Product6/1 -> Add3/2
  Product2/1 -> Add1/2
  Product1/1 -> Add1/1
  Add4/1 -> Gain3/1
  Gain3/1 -> Add5/2
  Constant1/1 -> Add5/1
  Add5/1 -> Trigonometric Function/2
  Add7/1 -> Trigonometric Function2/2
  Add6/1 -> Gain4/1
  Gain4/1 -> Add7/2
  Constant2/1 -> Add7/1
  Math Function2/1 -> Add4/1
  Math Function3/1 -> Add6/1, Add4/2
  Math Function4/1 -> Add6/2
  Demux/1 -> Add/1
  Demux/2 -> Add/2
  Demux/3 -> Add/3
  Demux/4 -> Add/4
  Math Function/1 -> Demux/1

== system MJAUV_Maneuverability_model_V2/MJ-AUV Model & PropulsionSystem/Dynamics and Kinematics/Subsystem6/Subsystem1/Subsystem ==
  "Euler Angles " : Inport
  Add : Sum
  Add1 : Sum  Inputs=-+
  Add2 : Sum
  Add3 : Sum  Inputs=+-
  Demux : Demux  Outputs=3
  Demux1 : Demux  Outputs=3
  Gain : Gain  Gain=0.5
  Mux : Mux
  Product{,1..7} (8 alike) : Product  Inputs=3
  Trigonometric Function : Trigonometry
  Trigonometric Function1 : Trigonometry  Operator=cos
  Quaternions : Outport  VectorParamsAs1DForOutWhenUnconnected=off
  wires:
  Add3/1 -> Mux/4
  Add2/1 -> Mux/3
  Add/1 -> Mux/1
  Add1/1 -> Mux/2
  Mux/1 -> Quaternions/1
  Product7/1 -> Add3/2
  Product6/1 -> Add3/1
  Product5/1 -> Add2/2
  Product4/1 -> Add2/1
  Product3/1 -> Add1/2
  Product2/1 -> Add1/1
  Product1/1 -> Add/2
  Product/1 -> Add/1
  Demux1/3 -> Product5/3, Product1/3, Product3/3, Product7/3  "cos(Y/2)"
  Demux1/1 -> Product5/1, Product2/1, Product1/1, Product6/1  "cos(R/2)"
  Demux1/2 -> Product6/2, Product1/2, Product3/2, Product4/2  "cos(P/2)"
  Trigonometric Function1/1 -> Demux1/1
  Demux/3 -> Product/3, Product2/3, Product4/3, Product6/3  "sin(Y/2)"
  Demux/2 -> Product/2, Product2/2, Product5/2, Product7/2  "sin(P/2)"
  Demux/1 -> Product/1, Product3/1, Product4/1, Product7/1  "sin(R/2)"
  Trigonometric Function/1 -> Demux/1
  Gain/1 -> Trigonometric Function/1, Trigonometric Function1/1
  "Euler Angles "/1 -> Gain/1

== system MJAUV_Maneuverability_model_V2/MJ-AUV Model & PropulsionSystem/Dynamics and Kinematics/Subsystem6/Subsystem1/Subsystem1 ==
  In2 : Inport
  Abs : Abs  SaturateOnIntegerOverflow=off
  Add : Sum  Inputs=-+
  Constant : Constant  Value=2*pi
  Switch : Switch  Criteria=u2 > Threshold  Threshold=pi  SaturateOnIntegerOverflow=off  InputSameDT=off
  Out1 : Outport
  wires:
  In2/1 -> Add/2, Switch/3, Abs/1
  Switch/1 -> Out1/1
  Add/1 -> Switch/1
  Abs/1 -> Switch/2
  Constant/1 -> Add/1

== system MJAUV_Maneuverability_model_V2/MJ-AUV Model & PropulsionSystem/Dynamics and Kinematics/Subsystem7/Added Mass Coriolis and centripetal matrix1/Skew Symmetrical Operator ==
  v : Inport
  Constant : Constant  Value=0
  Create 3x3 Matrix : sharedutil/Create 3x3 Matrix  aMode=aMode
  Demux : Demux  Outputs=3
      settings: DisplayOption=none
  Gain : Gain  Gain=-1  SaturateOnIntegerOverflow=on  OutDataTypeStr=Inherit: Same as input  ParamDataTypeStr=Inherit: Same as input
  Gain1 : Gain  Gain=-1  SaturateOnIntegerOverflow=on  OutDataTypeStr=Inherit: Same as input  ParamDataTypeStr=Inherit: Same as input
  Gain2 : Gain  Gain=-1  SaturateOnIntegerOverflow=on  OutDataTypeStr=Inherit: Same as input  ParamDataTypeStr=Inherit: Same as input
  S(V) : Outport  VectorParamsAs1DForOutWhenUnconnected=off
  wires:
  Constant/1 -> Create 3x3 Matrix/1, Create 3x3 Matrix/9, Create 3x3 Matrix/5
  Demux/1 -> Gain/1, Create 3x3 Matrix/8  "v(1)"
  Demux/2 -> Gain1/1, Create 3x3 Matrix/3  "v(2)"
  Demux/3 -> Gain2/1, Create 3x3 Matrix/4  "v(3)"
  Gain/1 -> Create 3x3 Matrix/6  "-v(1)"
  Gain1/1 -> Create 3x3 Matrix/7  "-v(2)"
  Gain2/1 -> Create 3x3 Matrix/2  "-v(3)"
  Create 3x3 Matrix/1 -> S(V)/1
  v/1 -> Demux/1

== system MJAUV_Maneuverability_model_V2/MJ-AUV Model & PropulsionSystem/Dynamics and Kinematics/Subsystem7/Added Mass Coriolis and centripetal matrix1/Skew Symmetrical Operator  ==
  v : Inport
  Constant : Constant  Value=0
  Create 3x3 Matrix : sharedutil/Create 3x3 Matrix  aMode=aMode
  Demux : Demux  Outputs=3
      settings: DisplayOption=none
  Gain : Gain  Gain=-1  SaturateOnIntegerOverflow=on  OutDataTypeStr=Inherit: Same as input  ParamDataTypeStr=Inherit: Same as input
  Gain1 : Gain  Gain=-1  SaturateOnIntegerOverflow=on  OutDataTypeStr=Inherit: Same as input  ParamDataTypeStr=Inherit: Same as input
  Gain2 : Gain  Gain=-1  SaturateOnIntegerOverflow=on  OutDataTypeStr=Inherit: Same as input  ParamDataTypeStr=Inherit: Same as input
  S(V) : Outport  VectorParamsAs1DForOutWhenUnconnected=off
  wires:
  v/1 -> Demux/1
  Create 3x3 Matrix/1 -> S(V)/1
  Gain2/1 -> Create 3x3 Matrix/2  "-v(3)"
  Gain1/1 -> Create 3x3 Matrix/7  "-v(2)"
  Gain/1 -> Create 3x3 Matrix/6  "-v(1)"
  Demux/3 -> Create 3x3 Matrix/4, Gain2/1  "v(3)"
  Demux/2 -> Create 3x3 Matrix/3, Gain1/1  "v(2)"
  Demux/1 -> Create 3x3 Matrix/8, Gain/1  "v(1)"
  Constant/1 -> Create 3x3 Matrix/5, Create 3x3 Matrix/9, Create 3x3 Matrix/1

== system MJAUV_Maneuverability_model_V2/MJ-AUV Model & PropulsionSystem/Dynamics and Kinematics/Subsystem7/Added Mass Coriolis and centripetal matrix1/Subsystem ==
  Create Diagonal Matrix1 : matrix_library/Create Diagonal Matrix
  K_pdot_T : Constant  Value=0
  M_qdot_T : Constant  Value=(pi*rho*R^2*LT^3)/12
  Mux : Mux  Inputs=6
  N_rdot_T : Constant  Value=(pi*rho*R^2*LT^3)/12
  Reshape1 : Reshape  OutputDimensionality=Column vector (2-D)  OutputDimensions=[6,6]
  X_udot_T : Constant  Value=0.1*mT
  Y_vdot_T : Constant  Value=pi*rho*R*R*LT
  Z_wdot_T : Constant  Value=pi*rho*R^2*LT
  MA_T : Outport
  wires:
  Z_wdot_T/1 -> Mux/3
  Mux/1 -> Reshape1/1
  Reshape1/1 -> Create Diagonal Matrix1/1
  Y_vdot_T/1 -> Mux/2
  X_udot_T/1 -> Mux/1
  M_qdot_T/1 -> Mux/5
  N_rdot_T/1 -> Mux/6
  K_pdot_T/1 -> Mux/4
  Create Diagonal Matrix1/1 -> MA_T/1

== system MJAUV_Maneuverability_model_V2/MJ-AUV Model & PropulsionSystem/Dynamics and Kinematics/Subsystem7/Restoring forces1/E1(e) ==
  e : Inport
  Gain : Gain  Gain=2  SaturateOnIntegerOverflow=on  OutDataTypeStr=Inherit: Same as input  ParamDataTypeStr=Inherit: Same as input
  "Gain " : Gain  Gain=2  SaturateOnIntegerOverflow=on  OutDataTypeStr=Inherit: Same as input  ParamDataTypeStr=Inherit: Same as input
  I (3x3) : Constant  Value=eye(3)
  Matrix Multiply : Product  Multiplication=Matrix(*)
  Product : Product  SaturateOnIntegerOverflow=on  OutDataTypeStr=Inherit: Same as first input
  Selector : Selector  InputPortWidth=4  IndexOptions=Index vector (dialog)  Indices=[1]  OutputSizes=1
  Selector1 : Selector  InputPortWidth=4  IndexOptions=Index vector (dialog)  Indices=[2 3 4]  OutputSizes=1
  Skew Symmetrical Operator : Subsystem
  Sum : Sum  Inputs=+++  SaturateOnIntegerOverflow=on
  E1 : Outport  VectorParamsAs1DForOutWhenUnconnected=off
  wires:
  e/1 -> Selector/1, Selector1/1
  Selector/1 -> "Gain "/1  "eta"
  Selector1/1 -> Skew Symmetrical Operator/1(v)  "eps"
  Skew Symmetrical Operator/1(S(V)) -> Matrix Multiply/1, Matrix Multiply/2, Product/2
  Matrix Multiply/1 -> Gain/1
  "Gain "/1 -> Product/1
  I (3x3)/1 -> Sum/1
  Product/1 -> Sum/2
  Gain/1 -> Sum/3
  Sum/1 -> E1/1
